simulink model "DPLL"  (R2020a)
settings: Solver=ode45  StartTime=0.0  StopTime=1e-3  RelTol=1e-3  EnableMultiTasking=on
libraries: simulink x5
settings Model: Creator=Tony  LastModifiedBy=Tony
settings DataIOCC: LimitDataPoints=on  SaveFormat=Array  ReturnWorkspaceOutputs=off
settings OptimizationCC: LifeSpan=inf
settings DebuggingCC: SolverPrmCheckMsg=warning  SFUnexpectedBacktrackingDiag=warning  SFNoUnconditionalDefaultTransitionDiag=warning  SFExecutionAtInitializationDiag=none  ArithmeticOperatorsInVariantConditions=warning
settings HardwareCC: ProdBitPerPointer=32  ProdBitPerSizeT=32  ProdBitPerPtrDiffT=32  ProdLargestAtomicFloat=None  ProdIntDivRoundTo=Undefined  ProdEndianess=Unspecified  ProdWordSize=32  ProdHWDeviceType=32-bit Generic
settings ModelReferenceCC: PropagateSignalLabelsOutOfModel=off
settings SFSimCC: SimUseLocalCustomCode=off  CustomCodeUndefinedFunction=UseInterfaceOnly
settings RTWCC: RTWUseLocalCustomCode=off
settings CodeAppCC: StateflowObjectComments=on
settings GRTTargetCC: TargetLangStandard=C89/C90 (ANSI)
settings ConfigComp: CovMetricSettings=dw  CovHtmlReporting=on  CovSaveCumulativeToWorkspaceVar=on  CovSaveSingleToWorkspaceVar=on  CovExternalEMLEnable=off  CovSFcnEnable=off

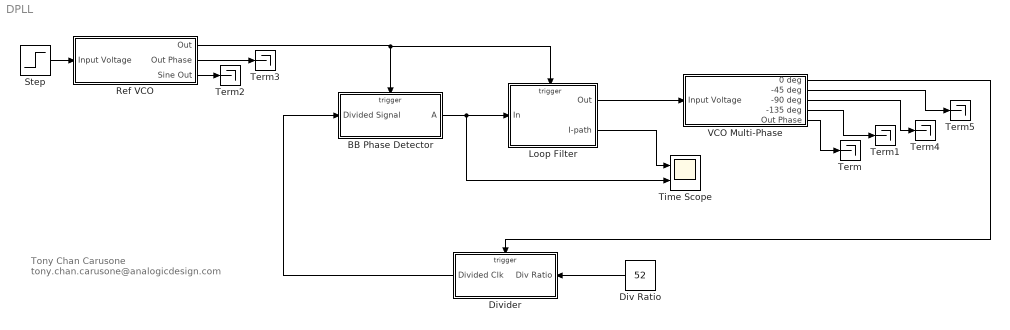
== system DPLL ==
  note: Tony Chan Carusone
      | tony.chan.carusone@analogicdesign.com
  BB Phase Detector : Subsystem
  Div Ratio : Constant  Value=52  OutDataTypeStr=int32
  Divider : Subsystem
  Loop Filter : Subsystem
  Ref VCO : Subsystem  mask{Kvco=20e6*2*pi, Ac=1, fo=0}
      mask prompts: fo "Default Frequency (fo)"
  Step : Step  Time=0  SampleTime=0
  Term{,1..5} (6 alike) : Terminator
  Time Scope : Scope  NumInputPorts=2
  VCO Multi-Phase : Subsystem  mask{Kvco=1e9*2*pi, fo=1000e6}
      mask prompts: fo "Default Frequency (fo)"
  wires:
  Divider/1(Divided Clk) -> BB Phase Detector/1(Divided Signal)
  VCO Multi-Phase/1(0 deg) -> Divider/Trigger
  Loop Filter/1(Out) -> VCO Multi-Phase/1(Input Voltage)
  Ref VCO/1(Out) -> Loop Filter/Trigger, BB Phase Detector/Trigger
  Step/1 -> Ref VCO/1(Input Voltage)
  Div Ratio/1 -> Divider/1(Div Ratio)
  VCO Multi-Phase/5(Out Phase) -> Term/1
  Ref VCO/3(Sine Out) -> Term2/1
  Ref VCO/2(Out Phase) -> Term3/1
  BB Phase Detector/1(A) -> Time Scope/2, Loop Filter/1(In)
  VCO Multi-Phase/4(-135 deg) -> Term1/1
  VCO Multi-Phase/3(-90 deg) -> Term4/1
  VCO Multi-Phase/2(-45 deg) -> Term5/1
  Loop Filter/2(I-path) -> Time Scope/1

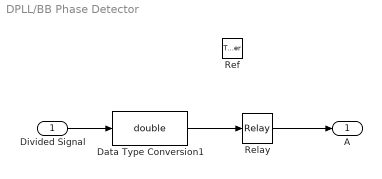
== system DPLL/BB Phase Detector ==
  Divided Signal : Inport
  Ref : TriggerPort  VariantControl=(inherit)
  Data Type Conversion1 : DataTypeConversion  OutDataTypeStr=double
  Relay : Relay  OffOutputValue=-1
  A : Outport
  wires:
  Relay/1 -> A/1
  Divided Signal/1 -> Data Type Conversion1/1
  Data Type Conversion1/1 -> Relay/1

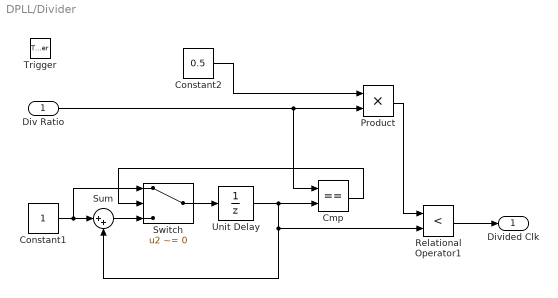
== system DPLL/Divider ==
  Div Ratio : Inport
  Trigger : TriggerPort  VariantControl=(inherit)
  Cmp : RelationalOperator  Operator===  OutDataTypeStr=boolean  RndMeth=Nearest
  Constant1 : Constant  OutDataTypeStr=int32
  Constant2 : Constant  Value=0.5
  Product : Product  RndMeth=Zero
  Relational Operator1 : RelationalOperator  Operator=<  OutDataTypeStr=boolean  RndMeth=Nearest
  Sum : Sum  Inputs=|++
  Switch : Switch  Criteria=u2 ~= 0
  Unit Delay : UnitDelay  SampleTime=-1  HasFrameUpgradeWarning=on
  Divided Clk : Outport
  wires:
  Constant1/1 -> Sum/1, Switch/1
  Sum/1 -> Switch/3
  Cmp/1 -> Switch/2
  Div Ratio/1 -> Cmp/1, Product/2
  Constant2/1 -> Product/1
  Product/1 -> Relational Operator1/1
  Relational Operator1/1 -> Divided Clk/1
  Unit Delay/1 -> Cmp/2, Relational Operator1/2, Sum/2
  Switch/1 -> Unit Delay/1

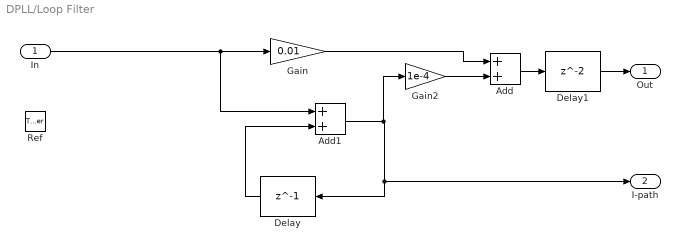
== system DPLL/Loop Filter ==
  In : Inport
  Ref : TriggerPort  VariantControl=(inherit)
  Add : Sum
  Add1 : Sum
  Delay : Delay  DelayLength=1  InitialCondition=0
  Delay1 : Delay  InitialCondition=0
  Gain : Gain  Gain=0.01
  Gain2 : Gain  Gain=1e-4
  Out : Outport
  I-path : Outport  Port=2
  wires:
  Delay/1 -> Add1/2
  Gain/1 -> Add/1
  Add1/1 -> Gain2/1, I-path/1, Delay/1
  Add/1 -> Delay1/1
  Delay1/1 -> Out/1
  Gain2/1 -> Add/2
  In/1 -> Add1/1, Gain/1

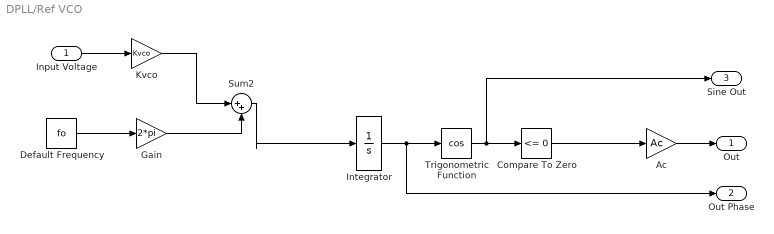
== system DPLL/Ref VCO ==
  Input Voltage : Inport
  Ac : Gain  Gain=Ac
  Compare To Zero : simulink/Logic and Bit Operations/Compare To Zero  relop=<=  OutDataTypeStr=uint8
  Default Frequency : Constant  Value=fo
  Gain : Gain  Gain=2*pi
  Integrator : Integrator
  Kvco : Gain  Gain=Kvco
  Sum2 : Sum  Inputs=|++
  Trigonometric Function : Trigonometry  Operator=cos
  Out : Outport
  Out Phase : Outport  Port=2
  Sine Out : Outport  Port=3
  wires:
  Ac/1 -> Out/1
  Compare To Zero/1 -> Ac/1
  Trigonometric Function/1 -> Sine Out/1, Compare To Zero/1
  Default Frequency/1 -> Gain/1
  Input Voltage/1 -> Kvco/1
  Integrator/1 -> Out Phase/1, Trigonometric Function/1
  Sum2/1 -> Integrator/1
  Gain/1 -> Sum2/2
  Kvco/1 -> Sum2/1

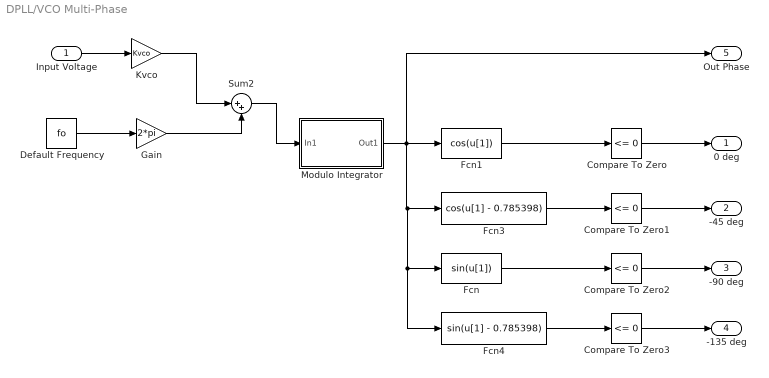
== system DPLL/VCO Multi-Phase ==
  Input Voltage : Inport
  Compare To Zero{,1..3} (4 alike) : simulink/Logic and Bit Operations/Compare To Zero  relop=<=  OutDataTypeStr=uint8
  Default Frequency : Constant  Value=fo
  Fcn : Fcn
  Fcn1 : Fcn  Expr=cos(u[1])
  Fcn3 : Fcn  Expr=cos(u[1] - 0.785398)
  Fcn4 : Fcn  Expr=sin(u[1] - 0.785398)
  Gain : Gain  Gain=2*pi
  Kvco : Gain  Gain=Kvco  OutDataTypeStr=Inherit: Inherit via back propagation
  Modulo Integrator : Subsystem
  Sum2 : Sum  Inputs=|++
  0 deg : Outport
  -45 deg : Outport  Port=2
  -90 deg : Outport  Port=3
  -135 deg : Outport  Port=4
  Out Phase : Outport  Port=5
  wires:
  Kvco/1 -> Sum2/1
  Gain/1 -> Sum2/2
  Sum2/1 -> Modulo Integrator/1(In1)
  Modulo Integrator/1(Out1) -> Fcn4/1, Fcn/1, Fcn3/1, Fcn1/1, Out Phase/1
  Input Voltage/1 -> Kvco/1
  Default Frequency/1 -> Gain/1
  Fcn4/1 -> Compare To Zero3/1
  Fcn3/1 -> Compare To Zero1/1
  Fcn1/1 -> Compare To Zero/1
  Fcn/1 -> Compare To Zero2/1
  Compare To Zero/1 -> 0 deg/1
  Compare To Zero1/1 -> -45 deg/1
  Compare To Zero2/1 -> -90 deg/1
  Compare To Zero3/1 -> -135 deg/1

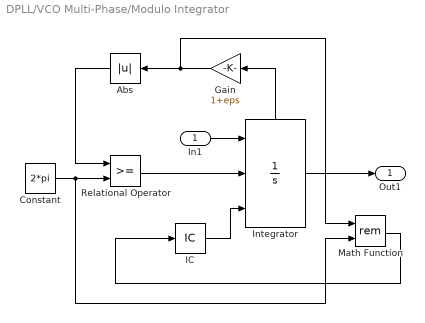
== system DPLL/VCO Multi-Phase/Modulo Integrator ==
  In1 : Inport
  Abs : Abs  SaturateOnIntegerOverflow=on
  Constant : Constant  Value=2*pi
  Gain : Gain  Gain=1+eps  SaturateOnIntegerOverflow=on  OutDataTypeStr=Inherit: Same as input  ParamDataTypeStr=Inherit: Same as input
  IC : InitialCondition  Value=0
  Integrator : Integrator  ExternalReset=rising  InitialConditionSource=external  UpperSaturationLimit=1  LowerSaturationLimit=0  ShowStatePort=on
  Math Function : Math  Operator=rem  SignedPower=on  SaturateOnIntegerOverflow=on
  Relational Operator : RelationalOperator  RndMeth=Nearest  InputSameDT=on
  Out1 : Outport
  wires:
  IC/1 -> Integrator/3
  In1/1 -> Integrator/1
  Integrator/1 -> Out1/1
  Math Function/1 -> IC/1
  Abs/1 -> Relational Operator/1
  Relational Operator/1 -> Integrator/2
  Constant/1 -> Math Function/2, Relational Operator/2
  Integrator/State -> Gain/1
  Gain/1 -> Abs/1, Math Function/1
